simulink model "MODE_5_COUNTER"  (R2020b)
settings: Solver=VariableStepAuto  StartTime=0.0  StopTime=inf  RelTol=1e-3
settings Model: PacingRate=1000  Creator=intel  LastModifiedBy=intel

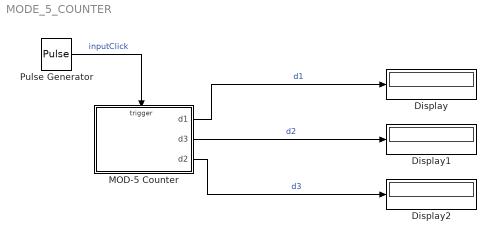
== system MODE_5_COUNTER ==
  Display : Display
  Display1 : Display
  Display2 : Display
  MOD-5 Counter : Stateflow chart  TreatAsAtomicUnit=on
  Pulse Generator : DiscretePulseGenerator  PulseType=Time based  Period=10  PulseWidth=5
  wires:
  MOD-5 Counter/1(d1) -> Display/1  "d1"
  MOD-5 Counter/2(d3) -> Display1/1  "d2"
  MOD-5 Counter/3(d2) -> Display2/1  "d3"
  Pulse Generator/1 -> MOD-5 Counter/Trigger  "inputClick"

== stateflow chart MODE_5_COUNTER/MOD-5 Counter ==
  settings: executeAtInitialization=1
  state digit1 [parallel]
    settings: executionOrder=1
    state two
      en: d1 = 2;
    state one
      en: d1 = 1;
    state three
      en:d1=3;
    state zero
      en: d1 = 0;
    state four
      en:d1=4;
    digit1.one -> digit1.two : inputClick
    digit1.two -> digit1.three : inputClick
    digit1.zero -> digit1.one : inputClick
    digit1.three -> digit1.four : inputClick
    digit1.four -> digit1.zero : inputClick /{digit2.inc2;}
    (default) -> digit1.zero
  state digit2 [parallel]
    settings: executionOrder=2
    state two
      en: d2 = 2;
    state one
      en: d2 = 1;
    state three
      en: d2=3;
    state zero
      en: d2 = 0;
    state four
      en: d2=4;
    digit2.one -> digit2.two : inc2
    digit2.zero -> digit2.one : inc2
    digit2.two -> digit2.three : inc2
    digit2.three -> digit2.four : inc2
    (default) -> digit2.zero
    digit2.four -> digit2.zero : inc2{digit3.inc3;}
  state digit3 [parallel]
    settings: executionOrder=3
    state three
      en: d3=3;
    state two
      en: d3 = 2;
    state one
      en: d3 = 1;
    state four
      en: d3=4;
    state zero
      en: d3 = 0;
    digit3.one -> digit3.two : inc3
    digit3.two -> digit3.three : inc3
    digit3.zero -> digit3.one : inc3
    digit3.three -> digit3.four : inc3
    digit3.four -> digit3.zero : inc3
    (default) -> digit3.zero
  data: d1 output; d3 output; d2 output
  events: inc2 local EITHER_EDGE_EVENT; inc3 local EITHER_EDGE_EVENT; inputClick input RISING_EDGE_EVENT
